simulink model "sim_5_twolink_force_control"  (R2021a)
settings: Solver=VariableStepAuto  StartTime=0.0  StopTime=15  MaxStep=1e-2
values from neighbouring files (symbols this model uses):
  b1 = 0.01    [sim_params.m]    (also in sim_params_force.m)
  b2 = 0.01    [sim_params.m]    (also in sim_params_force.m)
  D = [zeros(n); eye(n)]    [control_comparison_script.m]    (also in gen_twolink_ss.m = reshape([0.0,0.0,0.0,0.0,0.0,0.0,0.0,0.0],[4,2]))
  g = 9.80665    [sim_params.m]    (also in sim_params_force.m)
  L1x = 0.3    [sim_params.m]    (also in sim_params_force.m)
  L1y = 0.050    (= 0.05)    [sim_params.m]    (also in sim_params_force.m)
  L1z = 0.05    [sim_params.m]    (also in sim_params_force.m)
  L2x = 0.15    [sim_params.m]    (also in sim_params_force.m = 0.3)
  L2y = 0.05    [sim_params.m]    (also in sim_params_force.m)
  L2z = 0.05    [sim_params.m]    (also in sim_params_force.m)
  m1 = m1*1.25    [control_comparison_script.m]    (also in sim_params.m = 2.775; sim_params_force.m = 2.775)
  m2 = m2*1.25    [control_comparison_script.m]    (also in sim_params.m = 1.3875; sim_params_force.m = 2.775)
  max_joint_torque1 = 20    [sim_params.m]    (also in sim_params_force.m)
  max_joint_torque2 = 10    [sim_params.m]    (also in sim_params_force.m = 20)
undefined symbols (not defined in the file or in its folder): Da, KD, KD_a, Kd_p, Kd_p2, Kdt, KF, Kf_v, Kf_v2, KI, Ki_f, Ki_f2, Ki_p, Ki_p2, KP, KP_a, Kp_f, Kp_f2, Kp_p, Kp_p2, Levenberg, Ma, Marquardt, R_env, sigbuilder_block, W_env, X, Xenv, Y, Z
libraries: sm_lib x72, nesl_utility x58, pid_lib x14, simulink x3, robotmaniplib x2, robotcorelib x1
(part 5 of 6)

== system sim_5_twolink_force_control/Controller/Parallel Force//position control (stiff)/Force Controller ==
  note: PI force controllers
  Fd : Inport
  F : Inport  Port=2
  q : Inport  Port=3
  V : Inport  Port=4
  C_q1 : pid_lib/PID Controller (2DOF)  Controller=PI  Form=Parallel  TimeDomain=Continuous-time  UseExternalTs=off  SampleTime=-1  IntegratorMethod=Forward Euler  FilterMethod=Forward Euler  ControllerParametersSource=internal  P=KF(1)  I=KI(1)  D=Kdt(1)  UseFilter=on  N=100  b=1  c=1  TunerSelectOption=Transfer Function Based (PID Tuner App)  InitialConditionSource=internal  InitialConditionForIntegrator=0  InitialConditionForFilter=0  DifferentiatorICPrevScaledInput=0  ExternalReset=none  TrackingMode=off  Kt=1  LimitOutput=off  SatLimitsSource=internal  UpperSaturationLimit=max_joint_torque1  LowerSaturationLimit=-max_joint_torque1  LinearizeAsGain=on  AntiWindupMode=none  Kb=1  POutMin=[]  POutMax=[]  IOutMin=[]  IOutMax=[]  DOutMin=[]  DOutMax=[]  NOutMin=[]  NOutMax=[]  bOutMin=[]  bOutMax=[]  cOutMin=[]  cOutMax=[]  SumOutMin=[]  SumOutMax=[]  SaturationOutMin=[]  SaturationOutMax=[]  PParamMin=[]  PParamMax=[]  IParamMin=[]  IParamMax=[]  DParamMin=[]  DParamMax=[]  NParamMin=[]  NParamMax=[]  bParamMin=[]  bParamMax=[]  cParamMin=[]  cParamMax=[]  KbParamMin=[]  KbParamMax=[]  KtParamMin=[]  KtParamMax=[]  KbOutMin=[]  KbOutMax=[]  KtOutMin=[]  KtOutMax=[]  IntegratorOutMin=[]  IntegratorOutMax=[]  FilterOutMin=[]  FilterOutMax=[]  SumI1OutMin=[]  SumI1OutMax=[]  SumI2OutMin=[]  SumI2OutMax=[]  SumI3OutMin=[]  SumI3OutMax=[]  SumI4OutMin=[]  SumI4OutMax=[]  SumDOutMin=[]  SumDOutMax=[]  Sum1OutMin=[]  Sum1OutMax=[]  Sum2OutMin=[]  Sum2OutMax=[]  Sum3OutMin=[]  Sum3OutMax=[]  DifferentiatorOutMin=[]  DifferentiatorOutMax=[]  FilterDiffOutCoefMin=[]  FilterDiffOutCoefMax=[]  ReciprocalOutMin=[]  ReciprocalOutMax=[]  SumDenOutMin=[]  SumDenOutMax=[]  SumNumOutMin=[]  SumNumOutMax=[]  DivideOutMin=[]  DivideOutMax=[]  UdiffTsProdOutMin=[]  UdiffTsProdOutMax=[]  NTsProdOutMin=[]  NTsProdOutMax=[]  UintegralTsProdOutMin=[]  UintegralTsProdOutMax=[]  UngainTsProdOutMin=[]  UngainTsProdOutMax=[]  IntegratorContinuousStateAttributes=''  IntegratorStateMustResolveToSignalObject=off  IntegratorRTWStateStorageClass=Auto  FilterContinuousStateAttributes=''  FilterStateMustResolveToSignalObject=off  FilterRTWStateStorageClass=Auto  ParallelPVariant=InternalParameters  IdealPVariant=Disabled  IVariant=InternalParameters  DVariant=Disabled  bVariant=InternalParameters  cVariant=Disabled  IntegratorVariant=Continuous  SatVariant=Disabled  AWVariant=Passthrough  PCopyVariant=Disabled  TRVariant=Disabled  FdbkBlocksVariant=Forward  IdealPFdbkVariant=Disabled  SatFdbkVariant=Disabled  DerivativeFilterVariant=Disabled  NVariant=Disabled  NCopyVariant=Disabled_SignalSpec  FilterICVariant=Disabled  IntegratorICVariant=InternalICs  ExternalResetVariant=Disabled  TRSumVariant=Passthrough  SumFdbkVariant=Disabled  SumVariant=Sum_PI  TsampFilterVariant=InternalTs  TsampNgainVariant=Passthrough  TsampIntegralVariant=Passthrough  ExternalSaturationOutDataTypeStr=Inherit: Same as second input
      settings: SourceProductBaseCode=SL
  C_q2 : pid_lib/PID Controller (2DOF)  Controller=PI  Form=Parallel  TimeDomain=Continuous-time  UseExternalTs=off  SampleTime=-1  IntegratorMethod=Forward Euler  FilterMethod=Forward Euler  ControllerParametersSource=internal  P=KF(2)  I=KI(2)  D=Kdt(2)  UseFilter=on  N=100  b=1  c=1  TunerSelectOption=Transfer Function Based (PID Tuner App)  InitialConditionSource=internal  InitialConditionForIntegrator=0  InitialConditionForFilter=0  DifferentiatorICPrevScaledInput=0  ExternalReset=none  TrackingMode=off  Kt=1  LimitOutput=off  SatLimitsSource=internal  UpperSaturationLimit=max_joint_torque2  LowerSaturationLimit=-max_joint_torque2  LinearizeAsGain=on  AntiWindupMode=none  Kb=1  POutMin=[]  POutMax=[]  IOutMin=[]  IOutMax=[]  DOutMin=[]  DOutMax=[]  NOutMin=[]  NOutMax=[]  bOutMin=[]  bOutMax=[]  cOutMin=[]  cOutMax=[]  SumOutMin=[]  SumOutMax=[]  SaturationOutMin=[]  SaturationOutMax=[]  PParamMin=[]  PParamMax=[]  IParamMin=[]  IParamMax=[]  DParamMin=[]  DParamMax=[]  NParamMin=[]  NParamMax=[]  bParamMin=[]  bParamMax=[]  cParamMin=[]  cParamMax=[]  KbParamMin=[]  KbParamMax=[]  KtParamMin=[]  KtParamMax=[]  KbOutMin=[]  KbOutMax=[]  KtOutMin=[]  KtOutMax=[]  IntegratorOutMin=[]  IntegratorOutMax=[]  FilterOutMin=[]  FilterOutMax=[]  SumI1OutMin=[]  SumI1OutMax=[]  SumI2OutMin=[]  SumI2OutMax=[]  SumI3OutMin=[]  SumI3OutMax=[]  SumI4OutMin=[]  SumI4OutMax=[]  SumDOutMin=[]  SumDOutMax=[]  Sum1OutMin=[]  Sum1OutMax=[]  Sum2OutMin=[]  Sum2OutMax=[]  Sum3OutMin=[]  Sum3OutMax=[]  DifferentiatorOutMin=[]  DifferentiatorOutMax=[]  FilterDiffOutCoefMin=[]  FilterDiffOutCoefMax=[]  ReciprocalOutMin=[]  ReciprocalOutMax=[]  SumDenOutMin=[]  SumDenOutMax=[]  SumNumOutMin=[]  SumNumOutMax=[]  DivideOutMin=[]  DivideOutMax=[]  UdiffTsProdOutMin=[]  UdiffTsProdOutMax=[]  NTsProdOutMin=[]  NTsProdOutMax=[]  UintegralTsProdOutMin=[]  UintegralTsProdOutMax=[]  UngainTsProdOutMin=[]  UngainTsProdOutMax=[]  IntegratorContinuousStateAttributes=''  IntegratorStateMustResolveToSignalObject=off  IntegratorRTWStateStorageClass=Auto  FilterContinuousStateAttributes=''  FilterStateMustResolveToSignalObject=off  FilterRTWStateStorageClass=Auto  ParallelPVariant=InternalParameters  IdealPVariant=Disabled  IVariant=InternalParameters  DVariant=Disabled  bVariant=InternalParameters  cVariant=Disabled  IntegratorVariant=Continuous  SatVariant=Disabled  AWVariant=Passthrough  PCopyVariant=Disabled  TRVariant=Disabled  FdbkBlocksVariant=Forward  IdealPFdbkVariant=Disabled  SatFdbkVariant=Disabled  DerivativeFilterVariant=Disabled  NVariant=Disabled  NCopyVariant=Disabled_SignalSpec  FilterICVariant=Disabled  IntegratorICVariant=InternalICs  ExternalResetVariant=Disabled  TRSumVariant=Passthrough  SumFdbkVariant=Disabled  SumVariant=Sum_PI  TsampFilterVariant=InternalTs  TsampNgainVariant=Passthrough  TsampIntegralVariant=Passthrough  ExternalSaturationOutDataTypeStr=Inherit: Same as second input
      settings: SourceProductBaseCode=SL
  Demux : Demux  Outputs=2
  Demux1 : Demux  Outputs=2
  Mux : Mux  Inputs=2
  Scope : Scope  NumInputPorts=2
  Scope1 : Scope  NumInputPorts=2
  Scope5 : Scope
  Scope6 : Scope
  a_f : Outport
  wires:
  q/1 -> [PLANT]
  Fd/1 -> [Fd]
  F/1 -> [F]
  Demux/1 -> Scope/1, C_q1/1  "d"
  Demux1/1 -> Scope/2, C_q1/2
  Mux/1 -> a_f/1  "u_f"
  Demux/2 -> C_q2/1, Scope1/1  "d"
  Demux1/2 -> Scope1/2, C_q2/2
  C_q1/1 -> Scope5/1, Mux/1
  C_q2/1 -> Scope6/1, Mux/2
  [Fd] -> Demux/1  "F_desired"
  [F] -> Demux1/1  "Fs"
  V/1 -> [V]

== system sim_5_twolink_force_control/Controller/Parallel Force//position control (stiff)/Jacobian ==
  MODEL_BUS : Inport
  Bus Selector : BusSelector  OutputSignals=q1,q2
  Constant2 : Constant  Value=L1x
  Constant3 : Constant  Value=L2x
  Jacobian : MATLAB Function  TreatAsAtomicUnit=on
  J : Outport
  wires:
  Bus Selector/1 -> Jacobian/3(theta_1)  "<q1>"
  MODEL_BUS/1 -> Bus Selector/1
  Bus Selector/2 -> Jacobian/4(theta_2)  "<q2>"
  Constant3/1 -> Jacobian/2(L_2)
  Constant2/1 -> Jacobian/1(L_1)
  Jacobian/1(J) -> J/1  "J"

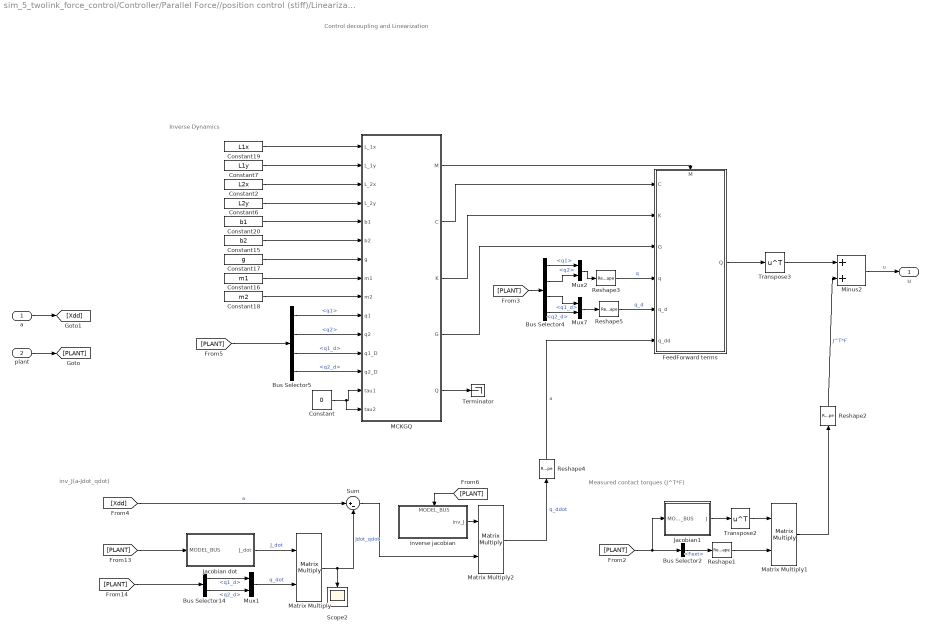
== system sim_5_twolink_force_control/Controller/Parallel Force//position control (stiff)/Linearization and decoupling ==
  note: Inverse Dynamics
  note: Measured contact torques (J^T*F)
  note: inv_J(a-Jdot_qdot)
  note: Control decoupling and Linearization
  a : Inport
  plant : Inport  Port=2
  Bus Selector14 : BusSelector  OutputSignals=q1_d,q2_d
  Bus Selector2 : BusSelector  OutputSignals=Fext
  Bus Selector4 : BusSelector  OutputSignals=q1,q2,q1_d,q2_d
  Bus Selector5 : BusSelector  OutputSignals=q1,q2,q1_d,q2_d
  Constant : Constant  Value=0
  Constant15 : Constant  Value=b2
  Constant16 : Constant  Value=m1
  Constant17 : Constant  Value=g
  Constant18 : Constant  Value=m2
  Constant19 : Constant  Value=L1x
  Constant2 : Constant  Value=L2x
  Constant20 : Constant  Value=b1
  Constant6 : Constant  Value=L2y
  Constant7 : Constant  Value=L1y
  FeedForward terms : Subsystem
      settings: PortSchema="{\"entries\":[{\"content\":{\"sides\":[{\"content\":{\"connectorIds\":[\"In1\",\"In2\",\"In3\",\"In4\",\"In5\",\"In6\"]},\"type\":\"ConnectorPlacement.EquallySpacedRectSide\",\"uuid\":\"236e7a2f-027c-4887-b3e9-bc0e11a59ec6\"},{\"content\":{\"connectorIds\":[\"Out1\"],\"side\":\"RIGHT\"},\"type\":\"ConnectorPlacement.EquallySpacedRectSide\",\"uuid\":\"0b727d96-7650-4ea0-95ac-5fb1bad7af10\"},{\"content\":{\"connectorIds\":[\"In7\"],\"side\":\"TOP\"},\"type\":\"ConnectorPlacement.EquallySpacedRectSide\",\"uuid\":\"19d9c8c6-ae7e-49b4-b718-472bd3040569\"},{\"content\":{\"connectorIds\":[],\"side\":\"BOTTOM\"},\"type\":\"ConnectorPlacement.EquallySpacedRectSide\",\"uuid\":\"734f5953-872d-4718-8798-69ea98da43e1\"}]},\"type\":\"ConnectorPlacement.EquallySpacedConnector\",\"uuid\":\"f4b93fea-e2dd-47f1-bf2a-cf2dec03adb9\"}],\"packageUris\":[\"http://schema.mathworks.com/mf0/Connector/R2020b\"],\"version\":\"1.0\"}"
  Jacobian dot : Subsystem
  Jacobian1 : Subsystem
  MCKGQ : MATLAB Function  TreatAsAtomicUnit=on
  Matrix Multiply : Product  Multiplication=Matrix(*)
  Matrix Multiply1 : Product  Multiplication=Matrix(*)
  Matrix Multiply2 : Product  Multiplication=Matrix(*)
  Minus2 : Sum
  Mux1 : Mux  Inputs=2
  Mux2 : Mux  Inputs=2
  Mux7 : Mux  Inputs=2
  Reshape{1,3..5} (4 alike) : Reshape  OutputDimensionality=Column vector (2-D)
  Reshape2 : Reshape  OutputDimensionality=Row vector (2-D)
  Scope2 : Scope
  Sum : Sum  Inputs=|+-
  Terminator : Terminator
  Transpose2 : Math  Operator=transpose  SaturateOnIntegerOverflow=on
  Transpose3 : Math  Operator=transpose  SaturateOnIntegerOverflow=on
  inverse jacobian : Subsystem
      settings: PortSchema="{\"entries\":[{\"content\":{\"sides\":[{\"content\":{\"connectorIds\":[]},\"type\":\"ConnectorPlacement.EquallySpacedRectSide\",\"uuid\":\"45ce6a23-782c-403d-9b70-ff0b21a50873\"},{\"content\":{\"connectorIds\":[\"Out1\"],\"side\":\"RIGHT\"},\"type\":\"ConnectorPlacement.EquallySpacedRectSide\",\"uuid\":\"4a96e012-75b5-4df2-9421-657ae1fb9404\"},{\"content\":{\"connectorIds\":[\"In1\"],\"side\":\"TOP\"},\"type\":\"ConnectorPlacement.EquallySpacedRectSide\",\"uuid\":\"9e57abfa-5fb6-4434-9322-f803ee7796b4\"}]},\"type\":\"ConnectorPlacement.EquallySpacedConnector\",\"uuid\":\"c3056cdb-9e74-460c-808f-59c03416937d\"}],\"packageUris\":[\"http://schema.mathworks.com/mf0/Connector/R2020b\"],\"version\":\"1.0\"}"
  u : Outport
  wires:
  Bus Selector2/1 -> Reshape1/1  "<Fext>"
  Constant19/1 -> MCKGQ/1(L_1x)
  MCKGQ/2(C) -> FeedForward terms/1(C)
  Bus Selector5/2 -> MCKGQ/11(q2)  "<q2>"
  Bus Selector4/3 -> Mux7/1  "<q1_d>"
  Reshape2/1 -> Minus2/2  "J^T*F"
  Transpose2/1 -> Matrix Multiply1/1
  Constant2/1 -> MCKGQ/3(L_2x)
  Reshape3/1 -> FeedForward terms/4(q)  "q"
  Bus Selector4/2 -> Mux2/2  "<q2>"
  Bus Selector5/4 -> MCKGQ/13(q2_D)  "<q2_d>"
  Mux2/1 -> Reshape3/1
  FeedForward terms/1(Q) -> Transpose3/1
  Bus Selector5/3 -> MCKGQ/12(q1_D)  "<q1_d>"
  Constant7/1 -> MCKGQ/2(L_1y)
  Constant6/1 -> MCKGQ/4(L_2y)
  Bus Selector4/4 -> Mux7/2  "<q2_d>"
  Bus Selector4/1 -> Mux2/1  "<q1>"
  Constant16/1 -> MCKGQ/8(m1)
  Bus Selector5/1 -> MCKGQ/10(q1)  "<q1>"
  MCKGQ/4(G) -> FeedForward terms/3(G)
  Constant18/1 -> MCKGQ/9(m2)
  Constant20/1 -> MCKGQ/5(b1)
  Constant15/1 -> MCKGQ/6(b2)
  Constant/1 -> MCKGQ/14(tau1), MCKGQ/15(tau2)
  Jacobian1/1(J) -> Transpose2/1
  Constant17/1 -> MCKGQ/7(g)
  [PLANT] -> Bus Selector5/1
  Matrix Multiply1/1 -> Reshape2/1
  Minus2/1 -> u/1  "u"
  MCKGQ/1(M) -> FeedForward terms/7(M)
  Mux7/1 -> Reshape5/1
  Reshape1/1 -> Matrix Multiply1/2
  Reshape5/1 -> FeedForward terms/5(q_d)  "q_d"
  MCKGQ/3(K) -> FeedForward terms/2(K)
  [PLANT] -> Bus Selector4/1
  [PLANT] -> Bus Selector2/1, Jacobian1/1(MODEL_BUS)
  Transpose3/1 -> Minus2/1
  plant/1 -> [PLANT]
  a/1 -> [Xdd]
  [PLANT] -> Jacobian dot/1(MODEL_BUS)
  [PLANT] -> Bus Selector14/1
  Bus Selector14/1 -> Mux1/1  "<q1_d>"
  Jacobian dot/1(J_dot) -> Matrix Multiply/1  "J_dot"
  Bus Selector14/2 -> Mux1/2  "<q2_d>"
  Mux1/1 -> Matrix Multiply/2  "q_dot"
  Matrix Multiply/1 -> Sum/2, Scope2/1  "Jdot_qdot"
  [Xdd] -> Sum/1  "a"
  [PLANT] -> inverse jacobian/1(MODEL_BUS)
  inverse jacobian/1(inv_J) -> Matrix Multiply2/1
  Sum/1 -> Matrix Multiply2/2
  Reshape4/1 -> FeedForward terms/6(q_dd)  "a"
  Matrix Multiply2/1 -> Reshape4/1  "q_ddot"
  MCKGQ/5(Q) -> Terminator/1

== system sim_5_twolink_force_control/Controller/Parallel Force//position control (stiff)/Position Controller ==
  X_d : Inport
  X : Inport  Port=2
  xdd : Inport  Port=3
  C_q1 : pid_lib/PID Controller (2DOF)  Controller=PD  Form=Parallel  TimeDomain=Continuous-time  UseExternalTs=off  SampleTime=-1  IntegratorMethod=Forward Euler  FilterMethod=Forward Euler  ControllerParametersSource=internal  P=KP(1)  I=Ki_p2(1)  D=KD(1)  UseFilter=on  N=100  b=1  c=1  TunerSelectOption=Transfer Function Based (PID Tuner App)  InitialConditionSource=internal  InitialConditionForIntegrator=0  InitialConditionForFilter=0  DifferentiatorICPrevScaledInput=0  ExternalReset=none  TrackingMode=off  Kt=1  LimitOutput=off  SatLimitsSource=internal  UpperSaturationLimit=max_joint_torque1  LowerSaturationLimit=-max_joint_torque1  LinearizeAsGain=on  AntiWindupMode=none  Kb=1  POutMin=[]  POutMax=[]  IOutMin=[]  IOutMax=[]  DOutMin=[]  DOutMax=[]  NOutMin=[]  NOutMax=[]  bOutMin=[]  bOutMax=[]  cOutMin=[]  cOutMax=[]  SumOutMin=[]  SumOutMax=[]  SaturationOutMin=[]  SaturationOutMax=[]  PParamMin=[]  PParamMax=[]  IParamMin=[]  IParamMax=[]  DParamMin=[]  DParamMax=[]  NParamMin=[]  NParamMax=[]  bParamMin=[]  bParamMax=[]  cParamMin=[]  cParamMax=[]  KbParamMin=[]  KbParamMax=[]  KtParamMin=[]  KtParamMax=[]  KbOutMin=[]  KbOutMax=[]  KtOutMin=[]  KtOutMax=[]  IntegratorOutMin=[]  IntegratorOutMax=[]  FilterOutMin=[]  FilterOutMax=[]  SumI1OutMin=[]  SumI1OutMax=[]  SumI2OutMin=[]  SumI2OutMax=[]  SumI3OutMin=[]  SumI3OutMax=[]  SumI4OutMin=[]  SumI4OutMax=[]  SumDOutMin=[]  SumDOutMax=[]  Sum1OutMin=[]  Sum1OutMax=[]  Sum2OutMin=[]  Sum2OutMax=[]  Sum3OutMin=[]  Sum3OutMax=[]  DifferentiatorOutMin=[]  DifferentiatorOutMax=[]  FilterDiffOutCoefMin=[]  FilterDiffOutCoefMax=[]  ReciprocalOutMin=[]  ReciprocalOutMax=[]  SumDenOutMin=[]  SumDenOutMax=[]  SumNumOutMin=[]  SumNumOutMax=[]  DivideOutMin=[]  DivideOutMax=[]  UdiffTsProdOutMin=[]  UdiffTsProdOutMax=[]  NTsProdOutMin=[]  NTsProdOutMax=[]  UintegralTsProdOutMin=[]  UintegralTsProdOutMax=[]  UngainTsProdOutMin=[]  UngainTsProdOutMax=[]  IntegratorContinuousStateAttributes=''  IntegratorStateMustResolveToSignalObject=off  IntegratorRTWStateStorageClass=Auto  FilterContinuousStateAttributes=''  FilterStateMustResolveToSignalObject=off  FilterRTWStateStorageClass=Auto  ParallelPVariant=InternalParameters  IdealPVariant=Disabled  IVariant=Disabled  DVariant=InternalParameters  bVariant=InternalParameters  cVariant=InternalParameters  IntegratorVariant=Disabled  SatVariant=Disabled  AWVariant=Disabled  PCopyVariant=Disabled  TRVariant=Disabled  FdbkBlocksVariant=Forward  IdealPFdbkVariant=Disabled  SatFdbkVariant=Disabled  DerivativeFilterVariant=ContFilter  NVariant=InternalParameters  NCopyVariant=Disabled  FilterICVariant=InternalICsFilter  IntegratorICVariant=Disabled  ExternalResetVariant=Disabled  TRSumVariant=Passthrough  SumFdbkVariant=Disabled  SumVariant=Sum_PD  TsampFilterVariant=InternalTs  TsampNgainVariant=Passthrough  TsampIntegralVariant=Disabled_SignalSpec  ExternalSaturationOutDataTypeStr=Inherit: Same as second input
      settings: SourceProductBaseCode=SL
  C_q2 : pid_lib/PID Controller (2DOF)  Controller=PD  Form=Parallel  TimeDomain=Continuous-time  UseExternalTs=off  SampleTime=-1  IntegratorMethod=Forward Euler  FilterMethod=Forward Euler  ControllerParametersSource=internal  P=KP(2)  I=Ki_p2(2)  D=KD(2)  UseFilter=on  N=100  b=1  c=1  TunerSelectOption=Transfer Function Based (PID Tuner App)  InitialConditionSource=internal  InitialConditionForIntegrator=0  InitialConditionForFilter=0  DifferentiatorICPrevScaledInput=0  ExternalReset=none  TrackingMode=off  Kt=1  LimitOutput=off  SatLimitsSource=internal  UpperSaturationLimit=max_joint_torque2  LowerSaturationLimit=-max_joint_torque2  LinearizeAsGain=on  AntiWindupMode=none  Kb=1  POutMin=[]  POutMax=[]  IOutMin=[]  IOutMax=[]  DOutMin=[]  DOutMax=[]  NOutMin=[]  NOutMax=[]  bOutMin=[]  bOutMax=[]  cOutMin=[]  cOutMax=[]  SumOutMin=[]  SumOutMax=[]  SaturationOutMin=[]  SaturationOutMax=[]  PParamMin=[]  PParamMax=[]  IParamMin=[]  IParamMax=[]  DParamMin=[]  DParamMax=[]  NParamMin=[]  NParamMax=[]  bParamMin=[]  bParamMax=[]  cParamMin=[]  cParamMax=[]  KbParamMin=[]  KbParamMax=[]  KtParamMin=[]  KtParamMax=[]  KbOutMin=[]  KbOutMax=[]  KtOutMin=[]  KtOutMax=[]  IntegratorOutMin=[]  IntegratorOutMax=[]  FilterOutMin=[]  FilterOutMax=[]  SumI1OutMin=[]  SumI1OutMax=[]  SumI2OutMin=[]  SumI2OutMax=[]  SumI3OutMin=[]  SumI3OutMax=[]  SumI4OutMin=[]  SumI4OutMax=[]  SumDOutMin=[]  SumDOutMax=[]  Sum1OutMin=[]  Sum1OutMax=[]  Sum2OutMin=[]  Sum2OutMax=[]  Sum3OutMin=[]  Sum3OutMax=[]  DifferentiatorOutMin=[]  DifferentiatorOutMax=[]  FilterDiffOutCoefMin=[]  FilterDiffOutCoefMax=[]  ReciprocalOutMin=[]  ReciprocalOutMax=[]  SumDenOutMin=[]  SumDenOutMax=[]  SumNumOutMin=[]  SumNumOutMax=[]  DivideOutMin=[]  DivideOutMax=[]  UdiffTsProdOutMin=[]  UdiffTsProdOutMax=[]  NTsProdOutMin=[]  NTsProdOutMax=[]  UintegralTsProdOutMin=[]  UintegralTsProdOutMax=[]  UngainTsProdOutMin=[]  UngainTsProdOutMax=[]  IntegratorContinuousStateAttributes=''  IntegratorStateMustResolveToSignalObject=off  IntegratorRTWStateStorageClass=Auto  FilterContinuousStateAttributes=''  FilterStateMustResolveToSignalObject=off  FilterRTWStateStorageClass=Auto  ParallelPVariant=InternalParameters  IdealPVariant=Disabled  IVariant=Disabled  DVariant=InternalParameters  bVariant=InternalParameters  cVariant=InternalParameters  IntegratorVariant=Disabled  SatVariant=Disabled  AWVariant=Disabled  PCopyVariant=Disabled  TRVariant=Disabled  FdbkBlocksVariant=Forward  IdealPFdbkVariant=Disabled  SatFdbkVariant=Disabled  DerivativeFilterVariant=ContFilter  NVariant=InternalParameters  NCopyVariant=Disabled  FilterICVariant=InternalICsFilter  IntegratorICVariant=Disabled  ExternalResetVariant=Disabled  TRSumVariant=Passthrough  SumFdbkVariant=Disabled  SumVariant=Sum_PD  TsampFilterVariant=InternalTs  TsampNgainVariant=Passthrough  TsampIntegralVariant=Disabled_SignalSpec  ExternalSaturationOutDataTypeStr=Inherit: Same as second input
      settings: SourceProductBaseCode=SL
  Demux : Demux  Outputs=2
  Demux1 : Demux  Outputs=2
  Mux : Mux  Inputs=2
  Scope : Scope  NumInputPorts=2
  Scope2 : Scope  NumInputPorts=2
  Sum : Sum  Inputs=++|
  a_p : Outport
  wires:
  xdd/1 -> [Xdd]
  X_d/1 -> [Xd]
  X/1 -> [X]
  C_q1/1 -> Mux/1
  C_q2/1 -> Mux/2
  [Xd] -> Demux/1  "Xs_desired"
  [X] -> Demux1/1  "Xs"
  Demux/1 -> C_q1/1, Scope/1  "d1"
  Demux/2 -> Scope2/1, C_q2/1  "d2"
  Demux1/1 -> Scope/2, C_q1/2
  Demux1/2 -> Scope2/2, C_q2/2
  Mux/1 -> Sum/2
  Sum/1 -> a_p/1
  [Xdd] -> Sum/1

== system sim_5_twolink_force_control/Controller/Parallel Force//position control (stiff)/Saturate Inputs ==
  inp : Inport
  Demux : Demux  Outputs=2
  Mux : Mux  Inputs=2
  Saturate Gripper Force : Saturate  UpperLimit=max_joint_torque2  LowerLimit=-max_joint_torque2
  Saturate Joint Torques : Saturate  UpperLimit=max_joint_torque1  LowerLimit=-max_joint_torque1
  sat : Outport  VectorParamsAs1DForOutWhenUnconnected=off
  wires:
  Saturate Joint Torques/1 -> Mux/1
  Demux/1 -> Saturate Joint Torques/1
  Mux/1 -> sat/1
  Saturate Gripper Force/1 -> Mux/2
  inp/1 -> Demux/1
  Demux/2 -> Saturate Gripper Force/1

== system sim_5_twolink_force_control/Robot+Environment/ARM+ Wall(complaint)  Simscape/Saturate Inputs ==
  inp : Inport
  Demux : Demux  Outputs=2
  Mux : Mux  Inputs=2
  Saturate Gripper Force : Saturate  UpperLimit=max_joint_torque2  LowerLimit=-max_joint_torque2
  Saturate Joint Torques : Saturate  UpperLimit=max_joint_torque1  LowerLimit=-max_joint_torque1
  sat : Outport  VectorParamsAs1DForOutWhenUnconnected=off
  wires:
  Saturate Joint Torques/1 -> Mux/1
  Demux/1 -> Saturate Joint Torques/1
  Mux/1 -> sat/1
  Saturate Gripper Force/1 -> Mux/2
  inp/1 -> Demux/1
  Demux/2 -> Saturate Gripper Force/1

== system sim_5_twolink_force_control/Robot+Environment/ARM+Wall(stiff) Simscape/Saturate Inputs ==
  inp : Inport
  Demux : Demux  Outputs=2
  Mux : Mux  Inputs=2
  Saturate Gripper Force : Saturate  UpperLimit=max_joint_torque2  LowerLimit=-max_joint_torque2
  Saturate Joint Torques : Saturate  UpperLimit=max_joint_torque1  LowerLimit=-max_joint_torque1
  sat : Outport  VectorParamsAs1DForOutWhenUnconnected=off
  wires:
  Saturate Joint Torques/1 -> Mux/1
  Demux/1 -> Saturate Joint Torques/1
  Mux/1 -> sat/1
  Saturate Gripper Force/1 -> Mux/2
  inp/1 -> Demux/1
  Demux/2 -> Saturate Gripper Force/1

== system sim_5_twolink_force_control/Robot+Environment/ARM+curve(stiff) Simscape/Saturate Inputs ==
  inp : Inport
  Demux : Demux  Outputs=2
  Mux : Mux  Inputs=2
  Saturate Gripper Force : Saturate  UpperLimit=max_joint_torque2  LowerLimit=-max_joint_torque2
  Saturate Joint Torques : Saturate  UpperLimit=max_joint_torque1  LowerLimit=-max_joint_torque1
  sat : Outport  VectorParamsAs1DForOutWhenUnconnected=off
  wires:
  Saturate Joint Torques/1 -> Mux/1
  Demux/1 -> Saturate Joint Torques/1
  Mux/1 -> sat/1
  Saturate Gripper Force/1 -> Mux/2
  inp/1 -> Demux/1
  Demux/2 -> Saturate Gripper Force/1

== system sim_5_twolink_force_control/Robot+Environment/ARM+extrude(stiff) Simscape/Saturate Inputs ==
  inp : Inport
  Demux : Demux  Outputs=2
  Mux : Mux  Inputs=2
  Saturate Gripper Force : Saturate  UpperLimit=max_joint_torque2  LowerLimit=-max_joint_torque2
  Saturate Joint Torques : Saturate  UpperLimit=max_joint_torque1  LowerLimit=-max_joint_torque1
  sat : Outport  VectorParamsAs1DForOutWhenUnconnected=off
  wires:
  Saturate Joint Torques/1 -> Mux/1
  Demux/1 -> Saturate Joint Torques/1
  Mux/1 -> sat/1
  Saturate Gripper Force/1 -> Mux/2
  inp/1 -> Demux/1
  Demux/2 -> Saturate Gripper Force/1

== system sim_5_twolink_force_control/Robot+Environment/ARM+no constraints Simscape/Saturate Inputs ==
  inp : Inport
  Demux : Demux  Outputs=2
  Mux : Mux  Inputs=2
  Saturate Gripper Force : Saturate  UpperLimit=max_joint_torque2  LowerLimit=-max_joint_torque2
  Saturate Joint Torques : Saturate  UpperLimit=max_joint_torque1  LowerLimit=-max_joint_torque1
  sat : Outport  VectorParamsAs1DForOutWhenUnconnected=off
  wires:
  Saturate Joint Torques/1 -> Mux/1
  Demux/1 -> Saturate Joint Torques/1
  Mux/1 -> sat/1
  Saturate Gripper Force/1 -> Mux/2
  inp/1 -> Demux/1
  Demux/2 -> Saturate Gripper Force/1

== system sim_5_twolink_force_control/Trajectory/rampFx-stepXY command/Signal Builder ==
  Demux : Demux  Tag=STV Demux  Outputs=1
      settings: DisplayOption=none
  FromWs : FromWorkspace  Tag=STV FromWs  VariableName=tuvar
      SigBuilderData=|
      | common.afterFinalStr = 'Extrapolate'
      | common.sampleTime = 0
      | dataSet.timeRange = [0 12]
      | dataSet.name = 'Group 1'
      | sbobj.Groups.Name = 'Group 1'
      | sbobj.Groups.Signals.Name = 'Signal 1'
      | sbobj.Groups.Signals.XData = [0 4 8.02 12]
      | sbobj.Groups.Signals.YData = [10 10 30 30]
      | sbobj.Groups.TimeRange = [0 12]
  Signal 1 : Outport  Tag=STV Outport
  wires:
  Demux/1 -> Signal 1/1
  FromWs/1 -> Demux/1

== system sim_5_twolink_force_control/Trajectory/rampFx-stepXY command/Signal Builder1 ==
  Demux : Demux  Tag=STV Demux  Outputs=1
      settings: DisplayOption=none
  FromWs : FromWorkspace  Tag=STV FromWs  VariableName=tuvar
      SigBuilderData=|
      | common.afterFinalStr = 'Extrapolate'
      | common.sampleTime = 0
      | dataSet.timeRange = [0 12]
      | dataSet.name = 'Group 1'
      | sbobj.Groups.Name = 'Group 1'
      | sbobj.Groups.Signals.Name = 'Signal 1'
      | sbobj.Groups.Signals.XData = [0 1.98 1.98 2 8.02 12]
      | sbobj.Groups.Signals.YData = [0.25 0.25 0.25 0.25 0.15 0.15]
      | sbobj.Groups.TimeRange = [0 12]
  Signal 1 : Outport  Tag=STV Outport
  wires:
  Demux/1 -> Signal 1/1
  FromWs/1 -> Demux/1

== system sim_5_twolink_force_control/Trajectory/stepF command/Signal Builder ==
  Demux : Demux  Tag=STV Demux  Outputs=1
      settings: DisplayOption=none
  FromWs : FromWorkspace  Tag=STV FromWs  VariableName=tuvar
      SigBuilderData=|
      | common.afterFinalStr = 'Extrapolate'
      | common.sampleTime = 0
      | dataSet.timeRange = [0 12]
      | dataSet.name = 'Group 1'
      | sbobj.Groups.Name = 'Group 1'
      | sbobj.Groups.Signals.Name = 'Signal 1'
      | sbobj.Groups.Signals.XData = [0 4 4 8.02 8.02 12]
      | sbobj.Groups.Signals.YData = [10 10 20 20 30 30]
      | sbobj.Groups.TimeRange = [0 12]
  Signal 1 : Outport  Tag=STV Outport
  wires:
  Demux/1 -> Signal 1/1
  FromWs/1 -> Demux/1

== system sim_5_twolink_force_control/Trajectory/stepF-stepXY command/Signal Builder ==
  Demux : Demux  Tag=STV Demux  Outputs=1
      settings: DisplayOption=none
  FromWs : FromWorkspace  Tag=STV FromWs  VariableName=tuvar
      SigBuilderData=|
      | common.afterFinalStr = 'Extrapolate'
      | common.sampleTime = 0
      | dataSet.timeRange = [0 12]
      | dataSet.name = 'Group 1'
      | sbobj.Groups.Name = 'Group 1'
      | sbobj.Groups.Signals.Name = 'Signal 1'
      | sbobj.Groups.Signals.XData = [0 4 4 8.02 8.02 12]
      | sbobj.Groups.Signals.YData = [10 10 20 20 30 30]
      | sbobj.Groups.TimeRange = [0 12]
  Signal 1 : Outport  Tag=STV Outport
  wires:
  Demux/1 -> Signal 1/1
  FromWs/1 -> Demux/1

== system sim_5_twolink_force_control/Trajectory/stepFx-rampY command/Signal Builder ==
  Demux : Demux  Tag=STV Demux  Outputs=1
      settings: DisplayOption=none
  FromWs : FromWorkspace  Tag=STV FromWs  VariableName=tuvar
      SigBuilderData=|
      | common.afterFinalStr = 'Extrapolate'
      | common.sampleTime = 0
      | dataSet.timeRange = [0 12]
      | dataSet.name = 'Group 1'
      | sbobj.Groups.Name = 'Group 1'
      | sbobj.Groups.Signals.Name = 'Signal 1'
      | sbobj.Groups.Signals.XData = [0 4 4 8.02 8.02 12]
      | sbobj.Groups.Signals.YData = [20 20 30 30 50 50]
      | sbobj.Groups.TimeRange = [0 12]
  Signal 1 : Outport  Tag=STV Outport
  wires:
  Demux/1 -> Signal 1/1
  FromWs/1 -> Demux/1

== system sim_5_twolink_force_control/Trajectory/stepFx-rampY command/Signal Builder1 ==
  Demux : Demux  Tag=STV Demux  Outputs=1
      settings: DisplayOption=none
  FromWs : FromWorkspace  Tag=STV FromWs  VariableName=tuvar
      SigBuilderData=|
      | common.afterFinalStr = 'Extrapolate'
      | common.sampleTime = 0
      | dataSet.timeRange = [0 12]
      | dataSet.name = 'Group 1'
      | sbobj.Groups.Name = 'Group 1'
      | sbobj.Groups.Signals.Name = 'Signal 1'
      | sbobj.Groups.Signals.XData = [0 1.98 1.98 2 8.02 12]
      | sbobj.Groups.Signals.YData = [0.25 0.25 0.25 0.25 0.15 0.15]
      | sbobj.Groups.TimeRange = [0 12]
  Signal 1 : Outport  Tag=STV Outport
  wires:
  Demux/1 -> Signal 1/1
  FromWs/1 -> Demux/1

== system sim_5_twolink_force_control/Controller/Admittance+Position control/Linearization and decoupling/FeedForward terms ==
  C : Inport
  K : Inport  Port=2
  G : Inport  Port=3
  q : Inport  Port=4
  q_d : Inport  Port=5
  q_dd : Inport  Port=6
  M : Inport  Port=7
  Product : Product  Multiplication=Matrix(*)
  Product2 : Product  Multiplication=Matrix(*)
  Product3 : Product  Multiplication=Matrix(*)
  Scope : Scope
  Sum : Sum  Inputs=+|+|+|+
  Q : Outport
  wires:
  K/1 -> Product/1
  Product/1 -> Sum/3
  Product2/1 -> Sum/1
  Sum/1 -> Q/1
  C/1 -> Product3/1
  Product3/1 -> Sum/2
  M/1 -> Product2/1
  q_dd/1 -> Product2/2
  q/1 -> Product/2
  q_d/1 -> Product3/2
  G/1 -> Scope/1, Sum/4

== system sim_5_twolink_force_control/Controller/Admittance+Position control/Linearization and decoupling/Jacobian dot ==
  MODEL_BUS : Inport
  " Jacobian dot" : MATLAB Function  TreatAsAtomicUnit=on
  Bus Selector : BusSelector  OutputSignals=q1,q2,q1_d,q2_d
  Constant2 : Constant  Value=L1x
  Constant3 : Constant  Value=L2x
  J_dot : Outport
  wires:
  " Jacobian dot"/1(J_dot) -> J_dot/1  "J_dot"
  Constant2/1 -> " Jacobian dot"/1(L_1)
  Constant3/1 -> " Jacobian dot"/2(L_2)
  Bus Selector/2 -> " Jacobian dot"/4(th2)  "<q2>"
  MODEL_BUS/1 -> Bus Selector/1
  Bus Selector/1 -> " Jacobian dot"/3(th1)  "<q1>"
  Bus Selector/3 -> " Jacobian dot"/5(th1_d)  "<q1_d>"
  Bus Selector/4 -> " Jacobian dot"/6(th2_d)  "<q2_d>"

== system sim_5_twolink_force_control/Controller/Admittance+Position control/Linearization and decoupling/inverse jacobian ==
  MODEL_BUS : Inport
  Bus Selector : BusSelector  OutputSignals=q1,q2
  Constant2 : Constant  Value=L1x
  Constant3 : Constant  Value=L2x
  Inverse Jacobian : MATLAB Function  TreatAsAtomicUnit=on
  inv_J : Outport
  wires:
  Inverse Jacobian/1(inv_J) -> inv_J/1  "inv_J"
  Constant2/1 -> Inverse Jacobian/1(L_1)
  Constant3/1 -> Inverse Jacobian/2(L_2)
  Bus Selector/2 -> Inverse Jacobian/4(th2)  "<q2>"
  MODEL_BUS/1 -> Bus Selector/1
  Bus Selector/1 -> Inverse Jacobian/3(th1)  "<q1>"

== system sim_5_twolink_force_control/Controller/Hybrid Force//position control /Force Controller/Force Projection ==
  q : Inport
  Bus Selector3 : BusSelector  OutputSignals=q1,q2
  Constant1 : Constant  Value=L2x
  Constant3 : Constant  Value=L1x
  Force projection (StJ_t) : MATLAB Function  TreatAsAtomicUnit=on
  P_force : Outport
  wires:
  Bus Selector3/2 -> Force projection (StJ_t)/4(theta_2)  "<q2>"
  Bus Selector3/1 -> Force projection (StJ_t)/3(theta_1)  "<q1>"
  Force projection (StJ_t)/1(StJ_t) -> P_force/1
  q/1 -> Bus Selector3/1
  Constant3/1 -> Force projection (StJ_t)/1(L_1)
  Constant1/1 -> Force projection (StJ_t)/2(L_2)

== system sim_5_twolink_force_control/Controller/Hybrid Force//position control /Force Controller/Force Projection1 ==
  q : Inport
  Bus Selector3 : BusSelector  OutputSignals=q1,q2
  Constant1 : Constant  Value=L2x
  Constant3 : Constant  Value=L1x
  Force projection (StJ_t) : MATLAB Function  TreatAsAtomicUnit=on
  P_force : Outport
  wires:
  Bus Selector3/2 -> Force projection (StJ_t)/4(theta_2)  "<q2>"
  Bus Selector3/1 -> Force projection (StJ_t)/3(theta_1)  "<q1>"
  Force projection (StJ_t)/1(StJ_t) -> P_force/1
  q/1 -> Bus Selector3/1
  Constant3/1 -> Force projection (StJ_t)/1(L_1)
  Constant1/1 -> Force projection (StJ_t)/2(L_2)

== system sim_5_twolink_force_control/Controller/Hybrid Force//position control /Force Controller/Force Projection2 ==
  q : Inport
  Bus Selector3 : BusSelector  OutputSignals=q1,q2
  Constant1 : Constant  Value=L2x
  Constant3 : Constant  Value=L1x
  Force projection (StJ_t) : MATLAB Function  TreatAsAtomicUnit=on
  P_force : Outport
  wires:
  Bus Selector3/2 -> Force projection (StJ_t)/4(theta_2)  "<q2>"
  Bus Selector3/1 -> Force projection (StJ_t)/3(theta_1)  "<q1>"
  Force projection (StJ_t)/1(StJ_t) -> P_force/1
  q/1 -> Bus Selector3/1
  Constant3/1 -> Force projection (StJ_t)/1(L_1)
  Constant1/1 -> Force projection (StJ_t)/2(L_2)

== system sim_5_twolink_force_control/Controller/Hybrid Force//position control /Force Controller/Saturate Inputs ==
  inp : Inport
  Demux : Demux  Outputs=2
  Mux : Mux  Inputs=2
  Saturate Gripper Force : Saturate  UpperLimit=max_joint_torque2  LowerLimit=-max_joint_torque2
  Saturate Joint Torques : Saturate  UpperLimit=max_joint_torque1  LowerLimit=-max_joint_torque1
  sat : Outport  VectorParamsAs1DForOutWhenUnconnected=off
  wires:
  Saturate Joint Torques/1 -> Mux/1
  Demux/1 -> Saturate Joint Torques/1
  Mux/1 -> sat/1
  Saturate Gripper Force/1 -> Mux/2
  inp/1 -> Demux/1
  Demux/2 -> Saturate Gripper Force/1

== system sim_5_twolink_force_control/Controller/Hybrid Force//position control /Position Controller1/Position Projection ==
  q : Inport
  Bus Selector3 : BusSelector  OutputSignals=q1,q2
  Constant1 : Constant  Value=L2x
  Constant3 : Constant  Value=L1x
  Position projection (SJ)+ : MATLAB Function  TreatAsAtomicUnit=on
  P_pos : Outport
  wires:
  Bus Selector3/2 -> Position projection (SJ)+/4(theta_2)  "<q2>"
  Bus Selector3/1 -> Position projection (SJ)+/3(theta_1)  "<q1>"
  Position projection (SJ)+/1(SJ_pinv) -> P_pos/1
  q/1 -> Bus Selector3/1
  Constant3/1 -> Position projection (SJ)+/1(L_1)
  Constant1/1 -> Position projection (SJ)+/2(L_2)

== system sim_5_twolink_force_control/Controller/Hybrid Force//position control /Position Controller1/Position Projection1 ==
  q : Inport
  Bus Selector3 : BusSelector  OutputSignals=q1,q2
  Constant1 : Constant  Value=L2x
  Constant3 : Constant  Value=L1x
  Position projection (SJ)+ : MATLAB Function  TreatAsAtomicUnit=on
  P_pos : Outport
  wires:
  Bus Selector3/2 -> Position projection (SJ)+/4(theta_2)  "<q2>"
  Bus Selector3/1 -> Position projection (SJ)+/3(theta_1)  "<q1>"
  Position projection (SJ)+/1(SJ_pinv) -> P_pos/1
  q/1 -> Bus Selector3/1
  Constant3/1 -> Position projection (SJ)+/1(L_1)
  Constant1/1 -> Position projection (SJ)+/2(L_2)

== system sim_5_twolink_force_control/Controller/Hybrid Force//position control /Position Controller1/Saturate Inputs ==
  inp : Inport
  Demux : Demux  Outputs=2
  Mux : Mux  Inputs=2
  Saturate Gripper Force : Saturate  UpperLimit=max_joint_torque2  LowerLimit=-max_joint_torque2
  Saturate Joint Torques : Saturate  UpperLimit=max_joint_torque1  LowerLimit=-max_joint_torque1
  sat : Outport  VectorParamsAs1DForOutWhenUnconnected=off
  wires:
  Saturate Joint Torques/1 -> Mux/1
  Demux/1 -> Saturate Joint Torques/1
  Mux/1 -> sat/1
  Saturate Gripper Force/1 -> Mux/2
  inp/1 -> Demux/1
  Demux/2 -> Saturate Gripper Force/1

== system sim_5_twolink_force_control/Controller/Hybrid Force//position control (stiff)/Force Controller/Force Projection ==
  q : Inport
  Bus Selector3 : BusSelector  OutputSignals=q1,q2
  Constant1 : Constant  Value=L2x
  Constant3 : Constant  Value=L1x
  Force projection (StJ_t) : MATLAB Function  TreatAsAtomicUnit=on
  P_force : Outport
  wires:
  Bus Selector3/2 -> Force projection (StJ_t)/4(theta_2)  "<q2>"
  Bus Selector3/1 -> Force projection (StJ_t)/3(theta_1)  "<q1>"
  Force projection (StJ_t)/1(StJ_t) -> P_force/1
  q/1 -> Bus Selector3/1
  Constant3/1 -> Force projection (StJ_t)/1(L_1)
  Constant1/1 -> Force projection (StJ_t)/2(L_2)

== system sim_5_twolink_force_control/Controller/Hybrid Force//position control (stiff)/Force Controller/Force Projection1 ==
  q : Inport
  Bus Selector3 : BusSelector  OutputSignals=q1,q2
  Constant1 : Constant  Value=L2x
  Constant3 : Constant  Value=L1x
  Force projection (StJ_t) : MATLAB Function  TreatAsAtomicUnit=on
  P_force : Outport
  wires:
  Bus Selector3/2 -> Force projection (StJ_t)/4(theta_2)  "<q2>"
  Bus Selector3/1 -> Force projection (StJ_t)/3(theta_1)  "<q1>"
  Force projection (StJ_t)/1(StJ_t) -> P_force/1
  q/1 -> Bus Selector3/1
  Constant3/1 -> Force projection (StJ_t)/1(L_1)
  Constant1/1 -> Force projection (StJ_t)/2(L_2)

== system sim_5_twolink_force_control/Controller/Hybrid Force//position control (stiff)/Force Controller/Force Projection2 ==
  q : Inport
  Bus Selector3 : BusSelector  OutputSignals=q1,q2
  Constant1 : Constant  Value=L2x
  Constant3 : Constant  Value=L1x
  Force projection (StJ_t) : MATLAB Function  TreatAsAtomicUnit=on
  P_force : Outport
  wires:
  Bus Selector3/2 -> Force projection (StJ_t)/4(theta_2)  "<q2>"
  Bus Selector3/1 -> Force projection (StJ_t)/3(theta_1)  "<q1>"
  Force projection (StJ_t)/1(StJ_t) -> P_force/1
  q/1 -> Bus Selector3/1
  Constant3/1 -> Force projection (StJ_t)/1(L_1)
  Constant1/1 -> Force projection (StJ_t)/2(L_2)

== system sim_5_twolink_force_control/Controller/Hybrid Force//position control (stiff)/Force Controller/Saturate Inputs ==
  inp : Inport
  Demux : Demux  Outputs=2
  Mux : Mux  Inputs=2
  Saturate Gripper Force : Saturate  UpperLimit=max_joint_torque2  LowerLimit=-max_joint_torque2
  Saturate Joint Torques : Saturate  UpperLimit=max_joint_torque1  LowerLimit=-max_joint_torque1
  sat : Outport  VectorParamsAs1DForOutWhenUnconnected=off
  wires:
  Saturate Joint Torques/1 -> Mux/1
  Demux/1 -> Saturate Joint Torques/1
  Mux/1 -> sat/1
  Saturate Gripper Force/1 -> Mux/2
  inp/1 -> Demux/1
  Demux/2 -> Saturate Gripper Force/1

== system sim_5_twolink_force_control/Controller/Hybrid Force//position control (stiff)/Position Controller1/Position Projection ==
  q : Inport
  Bus Selector3 : BusSelector  OutputSignals=q1,q2
  Constant1 : Constant  Value=L2x
  Constant3 : Constant  Value=L1x
  Position projection (SJ)+ : MATLAB Function  TreatAsAtomicUnit=on
  P_pos : Outport
  wires:
  Bus Selector3/2 -> Position projection (SJ)+/4(theta_2)  "<q2>"
  Bus Selector3/1 -> Position projection (SJ)+/3(theta_1)  "<q1>"
  Position projection (SJ)+/1(SJ_pinv) -> P_pos/1
  q/1 -> Bus Selector3/1
  Constant3/1 -> Position projection (SJ)+/1(L_1)
  Constant1/1 -> Position projection (SJ)+/2(L_2)

== system sim_5_twolink_force_control/Controller/Hybrid Force//position control (stiff)/Position Controller1/Position Projection1 ==
  q : Inport
  Bus Selector3 : BusSelector  OutputSignals=q1,q2
  Constant1 : Constant  Value=L2x
  Constant3 : Constant  Value=L1x
  Position projection (SJ)+ : MATLAB Function  TreatAsAtomicUnit=on
  P_pos : Outport
  wires:
  Bus Selector3/2 -> Position projection (SJ)+/4(theta_2)  "<q2>"
  Bus Selector3/1 -> Position projection (SJ)+/3(theta_1)  "<q1>"
  Position projection (SJ)+/1(SJ_pinv) -> P_pos/1
  q/1 -> Bus Selector3/1
  Constant3/1 -> Position projection (SJ)+/1(L_1)
  Constant1/1 -> Position projection (SJ)+/2(L_2)

== system sim_5_twolink_force_control/Controller/Hybrid Force//position control (stiff)/Position Controller1/Saturate Inputs ==
  inp : Inport
  Demux : Demux  Outputs=2
  Mux : Mux  Inputs=2
  Saturate Gripper Force : Saturate  UpperLimit=max_joint_torque2  LowerLimit=-max_joint_torque2
  Saturate Joint Torques : Saturate  UpperLimit=max_joint_torque1  LowerLimit=-max_joint_torque1
  sat : Outport  VectorParamsAs1DForOutWhenUnconnected=off
  wires:
  Saturate Joint Torques/1 -> Mux/1
  Demux/1 -> Saturate Joint Torques/1
  Mux/1 -> sat/1
  Saturate Gripper Force/1 -> Mux/2
  inp/1 -> Demux/1
  Demux/2 -> Saturate Gripper Force/1

== system sim_5_twolink_force_control/Controller/Parallel Force//position control (stiff)/Linearization and decoupling/FeedForward terms ==
  C : Inport
  K : Inport  Port=2
  G : Inport  Port=3
  q : Inport  Port=4
  q_d : Inport  Port=5
  q_dd : Inport  Port=6
  M : Inport  Port=7
  Product : Product  Multiplication=Matrix(*)
  Product2 : Product  Multiplication=Matrix(*)
  Product3 : Product  Multiplication=Matrix(*)
  Scope : Scope
  Sum : Sum  Inputs=+|+|+|+
  Q : Outport
  wires:
  K/1 -> Product/1
  Product/1 -> Sum/3
  Product2/1 -> Sum/1
  Sum/1 -> Q/1
  C/1 -> Product3/1
  Product3/1 -> Sum/2
  M/1 -> Product2/1
  q_dd/1 -> Product2/2
  q/1 -> Product/2
  q_d/1 -> Product3/2
  G/1 -> Scope/1, Sum/4

== system sim_5_twolink_force_control/Controller/Parallel Force//position control (stiff)/Linearization and decoupling/Jacobian dot ==
  MODEL_BUS : Inport
  " Jacobian dot" : MATLAB Function  TreatAsAtomicUnit=on
  Bus Selector : BusSelector  OutputSignals=q1,q2,q1_d,q2_d
  Constant2 : Constant  Value=L1x
  Constant3 : Constant  Value=L2x
  J_dot : Outport
  wires:
  " Jacobian dot"/1(J_dot) -> J_dot/1  "J_dot"
  Constant2/1 -> " Jacobian dot"/1(L_1)
  Constant3/1 -> " Jacobian dot"/2(L_2)
  Bus Selector/2 -> " Jacobian dot"/4(th2)  "<q2>"
  MODEL_BUS/1 -> Bus Selector/1
  Bus Selector/1 -> " Jacobian dot"/3(th1)  "<q1>"
  Bus Selector/3 -> " Jacobian dot"/5(th1_d)  "<q1_d>"
  Bus Selector/4 -> " Jacobian dot"/6(th2_d)  "<q2_d>"

== system sim_5_twolink_force_control/Controller/Parallel Force//position control (stiff)/Linearization and decoupling/Jacobian1 ==
  MODEL_BUS : Inport
  Bus Selector : BusSelector  OutputSignals=q1,q2
  Constant2 : Constant  Value=L1x
  Constant3 : Constant  Value=L2x
  Jacobian : MATLAB Function  TreatAsAtomicUnit=on
  J : Outport
  wires:
  Bus Selector/1 -> Jacobian/3(theta_1)  "<q1>"
  MODEL_BUS/1 -> Bus Selector/1
  Bus Selector/2 -> Jacobian/4(theta_2)  "<q2>"
  Constant3/1 -> Jacobian/2(L_2)
  Constant2/1 -> Jacobian/1(L_1)
  Jacobian/1(J) -> J/1  "J"

== system sim_5_twolink_force_control/Controller/Parallel Force//position control (stiff)/Linearization and decoupling/inverse jacobian ==
  MODEL_BUS : Inport
  Bus Selector : BusSelector  OutputSignals=q1,q2
  Constant2 : Constant  Value=L1x
  Constant3 : Constant  Value=L2x
  Inverse Jacobian : MATLAB Function  TreatAsAtomicUnit=on
  inv_J : Outport
  wires:
  Inverse Jacobian/1(inv_J) -> inv_J/1  "inv_J"
  Constant2/1 -> Inverse Jacobian/1(L_1)
  Constant3/1 -> Inverse Jacobian/2(L_2)
  Bus Selector/2 -> Inverse Jacobian/4(th2)  "<q2>"
  MODEL_BUS/1 -> Bus Selector/1
  Bus Selector/1 -> Inverse Jacobian/3(th1)  "<q1>"

== matlab function sim_5_twolink_force_control/Controller/Parallel Force//position control (stiff)/Linearization and decoupling/MCKGQ ==
  data: L_1x input; M output; L_1y input; L_2x input; L_2y input; b1 input; b2 input; g input; m1 input; m2 input; q1 input; q2 input; q1_D input; q2_D input; tau1 input; tau2 input; C output; K output; G output; Q output
function [M,C,K,G,Q] = MCKGQ(L_1x,L_1y,L_2x,L_2y,b1,b2,g,m1,m2,q1,q2,q1_D,q2_D,tau1,tau2)
%#codegen

%    This function was generated by the Symbolic Math Toolbox version 8.7.
%    30-May-2022 13:59:37

M = reshape([(L_1x.^2.*m1)./3.0+L_1x.^2.*m2+(L_1y.^2.*m1)./1.2e+1+(L_2x.^2.*m2)./4.0+L_1x.*L_2x.*m2.*cos(q2),(L_2x.*m2.*(L_2x+L_1x.*cos(q2).*2.0))./4.0,(L_2x.*m2.*(L_2x+L_1x.*cos(q2).*2.0))./4.0,(m2.*(L_2x.^2.*4.0+L_2y.^2))./1.2e+1],[2,2]);
if nargout > 1
    C = reshape([-L_1x.*L_2x.*m2.*q2_D.*sin(q2),(L_1x.*L_2x.*m2.*q1_D.*sin(q2))./2.0,L_1x.*L_2x.*m2.*q2_D.*sin(q2).*(-1.0./2.0),0.0],[2,2]);
end
if nargout > 2
    K = reshape([0.0,0.0,0.0,0.0],[2,2]);
end
if nargout > 3
    G = [(g.*(L_2x.*m2.*cos(q1+q2)+L_1x.*m1.*cos(q1)+L_1x.*m2.*cos(q1).*2.0))./2.0;(L_2x.*g.*m2.*cos(q1+q2))./2.0];
end
if nargout > 4
    Q = [tau1-b1.*q1_D;tau2-b2.*q2_D];
end

== matlab function sim_5_twolink_force_control/Controller/Parallel Force//position control (stiff)/Linearization and decoupling/inverse jacobian/Inverse Jacobian ==
  data: L_1 input; inv_J output; L_2 input; th1 input; th2 input
function inv_J = inv_jacobian(L_1,L_2,th1,th2)

inv_J = [
% [                            -cos(th1 + th2)/(L_1*cos(th1 + th2)*sin(th1) - L_1*sin(th1 + th2)*cos(th1)),                             -sin(th1 + th2)/(L_1*cos(th1 + th2)*sin(th1) - L_1*sin(th1 + th2)*cos(th1))];
% [(L_2*cos(th1 + th2) + L_1*cos(th1))/(L_1*L_2*cos(th1 + th2)*sin(th1) - L_1*L_2*sin(th1 + th2)*cos(th1)), (L_2*sin(th1 + th2) + L_1*sin(th1))/(L_1*L_2*cos(th1 + th2)*sin(th1) - L_1*L_2*sin(th1 + th2)*cos(th1))];
[                          cos(th1 + th2)/(L_1*sin(th2)),                           sin(th1 + th2)/(L_1*sin(th2))];
[-(L_2*cos(th1 + th2) + L_1*cos(th1))/(L_1*L_2*sin(th2)), -(L_2*sin(th1 + th2) + L_1*sin(th1))/(L_1*L_2*sin(th2))];
];

== matlab function sim_5_twolink_force_control/Inverse Kinmatics/IK/Inverse Kinematics ==
  data: x input; q1 output; y input; L1 input; L2 input; q2 output
function [q1, q2]= ik_rr(x,y,L1,L2)
%IK_RR 


tmp = (x^2+y^2-L1^2-L2^2)/(2*L1*L2);
if abs(tmp-1)<0.0001
    tmp = 1;
end

if abs(tmp)>1
    q2=0;
else
    q2 = acos(tmp);
    if isnan(q2) || isinf(q2) || ~isreal(q2)
        q2 = 0;
    end
end

q1 = atan2(y,x)-atan2(L2*sin(q2), L1+L2*cos(q2));
if isnan(q1) || isinf(q1) || ~isreal(q1)
    q1 = 0;
end

== matlab function sim_5_twolink_force_control/Controller/Admittance+Position control/Jacobian/Jacobian ==
  data: L_1 input; J output; L_2 input; theta_1 input; theta_2 input
function J = jacobian_geom(L_1,L_2,theta_1,theta_2)

J = [
       -L_1.*sin(theta_1)-L_2.*sin(theta_1+theta_2) , -L_2.*sin(theta_1+theta_2) ;
        L_1.*cos(theta_1)+L_2.*cos(theta_1+theta_2) ,  L_2.*cos(theta_1+theta_2) ;
    ];

== matlab function sim_5_twolink_force_control/Controller/Parallel Force//position control (stiff)/Jacobian/Jacobian ==
  data: L_1 input; J output; L_2 input; theta_1 input; theta_2 input
function J = jacobian_geom(L_1,L_2,theta_1,theta_2)

J = [
       -L_1.*sin(theta_1)-L_2.*sin(theta_1+theta_2) , -L_2.*sin(theta_1+theta_2) ;
        L_1.*cos(theta_1)+L_2.*cos(theta_1+theta_2) ,  L_2.*cos(theta_1+theta_2) ;
    ];

== matlab function sim_5_twolink_force_control/Controller/Admittance+Position control/Linearization and decoupling/Jacobian dot/ Jacobian dot ==
  data: L_1 input; J_dot output; L_2 input; th1 input; th2 input; th1_d input; th2_d input
function J_dot = jacobian_dot(L_1,L_2,th1,th2,th1_d, th2_d)

J_dot = [
    [- L_2*cos(th1 + th2)*(th1_d + th2_d) - L_1*th1_d*cos(th1), -L_2*cos(th1 + th2)*(th1_d + th2_d)];
    [- L_1*th1_d*sin(th1) - L_2*sin(th1 + th2)*(th1_d + th2_d), -L_2*sin(th1 + th2)*(th1_d + th2_d)];
];

== matlab function sim_5_twolink_force_control/Forward Kinmatics/Forward Kinematics ==
  data: L_1 input; XE output; L_2 input; theta_1 input; theta_2 input; YE output
function [XE,YE] = FK(L_1,L_2,theta_1,theta_2)

XE = L_2.*cos(theta_1+theta_2)+L_1.*cos(theta_1);
if nargout > 1
    YE = L_2.*sin(theta_1+theta_2)+L_1.*sin(theta_1);
end

== matlab function sim_5_twolink_force_control/Controller/Parallel Force//position control (stiff)/Linearization and decoupling/Jacobian dot/ Jacobian dot ==
  data: L_1 input; J_dot output; L_2 input; th1 input; th2 input; th1_d input; th2_d input
function J_dot = jacobian_dot(L_1,L_2,th1,th2,th1_d, th2_d)

J_dot = [
    [- L_2*cos(th1 + th2)*(th1_d + th2_d) - L_1*th1_d*cos(th1), -L_2*cos(th1 + th2)*(th1_d + th2_d)];
    [- L_1*th1_d*sin(th1) - L_2*sin(th1 + th2)*(th1_d + th2_d), -L_2*sin(th1 + th2)*(th1_d + th2_d)];
];

== matlab function sim_5_twolink_force_control/Forward Kinmatics/Jacobian dot1/ Jacobian dot ==
  data: L_1 input; J_dot output; L_2 input; th1 input; th2 input; th1_d input; th2_d input
function J_dot = jacobian_dot(L_1,L_2,th1,th2,th1_d, th2_d)

J_dot = [
    [- L_2*cos(th1 + th2)*(th1_d + th2_d) - L_1*th1_d*cos(th1), -L_2*cos(th1 + th2)*(th1_d + th2_d)];
    [- L_1*th1_d*sin(th1) - L_2*sin(th1 + th2)*(th1_d + th2_d), -L_2*sin(th1 + th2)*(th1_d + th2_d)];
];

== matlab function sim_5_twolink_force_control/Controller/Admittance+Position control/Linearization and decoupling/MCKGQ ==
  data: L_1x input; M output; L_1y input; L_2x input; L_2y input; b1 input; b2 input; g input; m1 input; m2 input; q1 input; q2 input; q1_D input; q2_D input; tau1 input; tau2 input; C output; K output; G output; Q output
function [M,C,K,G,Q] = MCKGQ(L_1x,L_1y,L_2x,L_2y,b1,b2,g,m1,m2,q1,q2,q1_D,q2_D,tau1,tau2)
%#codegen

%    This function was generated by the Symbolic Math Toolbox version 8.7.
%    30-May-2022 13:59:37

M = reshape([(L_1x.^2.*m1)./3.0+L_1x.^2.*m2+(L_1y.^2.*m1)./1.2e+1+(L_2x.^2.*m2)./4.0+L_1x.*L_2x.*m2.*cos(q2),(L_2x.*m2.*(L_2x+L_1x.*cos(q2).*2.0))./4.0,(L_2x.*m2.*(L_2x+L_1x.*cos(q2).*2.0))./4.0,(m2.*(L_2x.^2.*4.0+L_2y.^2))./1.2e+1],[2,2]);
if nargout > 1
    C = reshape([-L_1x.*L_2x.*m2.*q2_D.*sin(q2),(L_1x.*L_2x.*m2.*q1_D.*sin(q2))./2.0,L_1x.*L_2x.*m2.*q2_D.*sin(q2).*(-1.0./2.0),0.0],[2,2]);
end
if nargout > 2
    K = reshape([0.0,0.0,0.0,0.0],[2,2]);
end
if nargout > 3
    G = [(g.*(L_2x.*m2.*cos(q1+q2)+L_1x.*m1.*cos(q1)+L_1x.*m2.*cos(q1).*2.0))./2.0;(L_2x.*g.*m2.*cos(q1+q2))./2.0];
end
if nargout > 4
    Q = [tau1-b1.*q1_D;tau2-b2.*q2_D];
end

== matlab function sim_5_twolink_force_control/Controller/Admittance+Position control/Linearization and decoupling/inverse jacobian/Inverse Jacobian ==
  data: L_1 input; inv_J output; L_2 input; th1 input; th2 input
function inv_J = inv_jacobian(L_1,L_2,th1,th2)

inv_J = [
% [                            -cos(th1 + th2)/(L_1*cos(th1 + th2)*sin(th1) - L_1*sin(th1 + th2)*cos(th1)),                             -sin(th1 + th2)/(L_1*cos(th1 + th2)*sin(th1) - L_1*sin(th1 + th2)*cos(th1))];
% [(L_2*cos(th1 + th2) + L_1*cos(th1))/(L_1*L_2*cos(th1 + th2)*sin(th1) - L_1*L_2*sin(th1 + th2)*cos(th1)), (L_2*sin(th1 + th2) + L_1*sin(th1))/(L_1*L_2*cos(th1 + th2)*sin(th1) - L_1*L_2*sin(th1 + th2)*cos(th1))];
[                          cos(th1 + th2)/(L_1*sin(th2)),                           sin(th1 + th2)/(L_1*sin(th2))];
[-(L_2*cos(th1 + th2) + L_1*cos(th1))/(L_1*L_2*sin(th2)), -(L_2*sin(th1 + th2) + L_1*sin(th1))/(L_1*L_2*sin(th2))];
];

== matlab function sim_5_twolink_force_control/Inverse Kinmatics/Forward Kinmatics/Forward Kinematics ==
  data: L_1 input; XE output; L_2 input; theta_1 input; theta_2 input; YE output
function [XE,YE] = FK(L_1,L_2,theta_1,theta_2)

XE = L_2.*cos(theta_1+theta_2)+L_1.*cos(theta_1);
if nargout > 1
    YE = L_2.*sin(theta_1+theta_2)+L_1.*sin(theta_1);
end

== matlab function sim_5_twolink_force_control/Forward Kinmatics/Jacobian1 ==
  data: L_1 input; J output; L_2 input; theta_1 input; theta_2 input
function J = jacobian_geom(L_1,L_2,theta_1,theta_2)

J = [
       -L_1.*sin(theta_1)-L_2.*sin(theta_1+theta_2) , -L_2.*sin(theta_1+theta_2) ;
        L_1.*cos(theta_1)+L_2.*cos(theta_1+theta_2) ,  L_2.*cos(theta_1+theta_2) ;
    ];

== matlab function sim_5_twolink_force_control/Controller/Parallel Force//position control (stiff)/Linearization and decoupling/Jacobian1/Jacobian ==
  data: L_1 input; J output; L_2 input; theta_1 input; theta_2 input
function J = jacobian_geom(L_1,L_2,theta_1,theta_2)

J = [
       -L_1.*sin(theta_1)-L_2.*sin(theta_1+theta_2) , -L_2.*sin(theta_1+theta_2) ;
        L_1.*cos(theta_1)+L_2.*cos(theta_1+theta_2) ,  L_2.*cos(theta_1+theta_2) ;
    ];

== matlab function sim_5_twolink_force_control/Controller/Hybrid Force//position control /Force Controller/Force Projection/Force projection (StJ_t) ==
  data: L_1 input; L_2 input; StJ_t output; theta_1 input; theta_2 input
function StJ_t = P_force(L_1,L_2,theta_1,theta_2)
% Force projection (StJ_t)
% StJ_t = transpose((1-S)*J)

% force control in X axis
StJ_t = [
    [- L_1*sin(theta_1) - L_2*sin(theta_1 + theta_2), 0]
    [                    -L_2*sin(theta_1 + theta_2), 0]
];

% no force control at all

% StJ_t = [
%     0   0;
%     0   0;
% ];
